simulink subsystem "VehicleForTest_refsub"  (R2022a)
settings: Solver=VariableStepAuto  StartTime=0.0  StopTime=10.0  RelTol=1e-3
undefined symbols (not defined in the file): testharness
libraries: fl_lib x4, nesl_utility x2
settings Model: Creator=isaacito  LastModifiedBy=isaacito
settings SolverCC: AlgebraicLoopSolver=TrustRegion
settings DebuggingCC: UnconnectedInputMsg=warning  UnconnectedOutputMsg=warning  UnconnectedLineMsg=warning  SFMachineParentedDataDiag=warning
settings RTWCC: DLArmComputeVersion=19.05

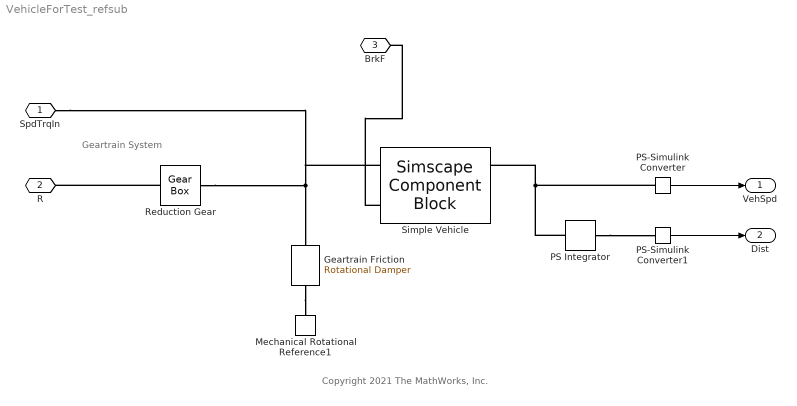
== system VehicleForTest_refsub ==
  note: Geartrain System
  note: Copyright 2021 The MathWorks, Inc.
  Geartrain Friction : fl_lib/Mechanical/Rotational Elements/Rotational Damper  D=testharness.geartrainFriction_Nm_per_rpm m*N/rpm  w_specify=off  w_priority=None  w=0 rad/s  w_nominal_specify=off  w_nominal_unit=rad/s  w_nominal_value=1  t_specify=off  t_priority=None  t=0 N*m  t_nominal_specify=off  t_nominal_unit=N*m  t_nominal_value=1
      settings: SourceProductBaseCode=PW,SS,VE
      settings: AttributesFormatString=|
      | %<D>
      | %<D_unit>
  Mechanical Rotational Reference1 : fl_lib/Mechanical/Rotational Elements/Mechanical Rotational Reference
      settings: SourceProductBaseCode=PW,SS,VE
  PS Integrator : fl_lib/Physical Signals/Linear Operators/PS Integrator  reset_method=foundation.enum.IntegratorResetSpec.None  initial_condition_spec=foundation.enum.IntegratorICSpec.Internal  x0=0 km
      settings: SourceProductBaseCode=PW,SS,VE
      settings: AttributesFormatString=|
      | Initial: %<x0>
      | Unit: %<x0_unit>
  PS-Simulink Converter : nesl_utility/PS-Simulink Converter  PhysicalDomain=network_engine_domain  SubClassName=ps_output  LeftPortType=input  RightPortType=output  PseudoPeriodic=off  Frequencies=[]  VectorFormat=1-D array  Unit=km/hr  AffineConversion=off
      settings: SourceProductBaseCode=SS,PW,VE
  PS-Simulink Converter1 : nesl_utility/PS-Simulink Converter  PhysicalDomain=network_engine_domain  SubClassName=ps_output  LeftPortType=input  RightPortType=output  PseudoPeriodic=off  Frequencies=[]  VectorFormat=1-D array  Unit=km  AffineConversion=off
      settings: SourceProductBaseCode=SS,PW,VE
  Reduction Gear : fl_lib/Mechanical/Mechanisms/Gear Box  ratio=testharness.reducerGearRatio_1  t_in_specify=off  t_in_priority=None  t_in=0 N*m  t_in_nominal_specify=off  t_in_nominal_unit=N*m  t_in_nominal_value=1  t_out_specify=off  t_out_priority=None  t_out=0 N*m  t_out_nominal_specify=off  t_out_nominal_unit=N*m  t_out_nominal_value=1
      settings: AttributesFormatString=%<ratio>  SourceProductBaseCode=PW,SS,VE
  Simple Vehicle : SimscapeComponentBlock  SourceFile=SimpleVehicle  ComponentPath=SimpleVehicle  ComponentVariants="[\"SimpleVehicle\"]"  ComponentVariantNames="[\"SimpleVehicle\"]"  ClassName=SimpleVehicle  SchemaVersion=1  R=testharness.tireRollingRadius_m m  M=testharness.vehicleMass_kg kg  v_specify=off  v_priority=High  v=0 km/hr  v_nominal_specify=off  v_nominal_unit=km/hr  v_nominal_value=1
      settings: CopyFcn=simscape.engine.sli.internal.componentblockcallback(gcbh,'COPY')  PreCopyFcn=simscape.engine.sli.internal.componentblockcallback(gcbh,'PRECOPY')  PreDeleteFcn=simscape.engine.sli.internal.componentblockcallback(gcbh,'PREDELETE')  InternalSimscapePortConfiguration="{\"Bottom\":[],\"Left\":[{\"id\":\"Axle\",\"label\":\"Axle\",\"type\":\"foundation.mechanical.rotational.rotational\"}],\"Right\":[{\"id\":\"V_out\",\"label\":\"V\",\"type\":\"output\"},{\"id\":\"Pwr\",\"label\":\"Pwr\",\"type\":\"output\"}],\"Top\":[{\"id\":\"BrkF\",\"label\":\"BrkF\",\"type\":\"input\"}]}"
      settings: AttributesFormatString=|
      | %<R>
      | %<M>
      mask Type: Rudimentary Longitudinal Vehicle
  SpdTrqIn : PMIOPort  Side=Left
  R : PMIOPort  Port=2  Side=Left
  BrkF : PMIOPort  Port=3  Side=Left
  VehSpd : Outport
  Dist : Outport  Port=2
  wires:
  PS-Simulink Converter/1 -> VehSpd/1
  PS-Simulink Converter1/1 -> Dist/1
  connections:
  Reduction Gear/RConn1 -- SpdTrqIn/RConn1 -- Simple Vehicle/LConn1 -- Geartrain Friction/LConn1
  PS-Simulink Converter/LConn1 -- PS Integrator/LConn1 -- Simple Vehicle/RConn1
  Reduction Gear/LConn1 -- R/RConn1
  Geartrain Friction/RConn1 -- Mechanical Rotational Reference1/LConn1
  Simple Vehicle/LConn2 -- BrkF/RConn1
  PS Integrator/RConn1 -- PS-Simulink Converter1/LConn1
